simulink subsystem "contact_cana"  (R2024a)
settings: Solver=VariableStepAuto  StartTime=0.0  StopTime=10.0  RelTol=1e-3
libraries: nesl_utility x12, sm_lib x12
settings Model: Creator=Acwa-Remote  LastModifiedBy=VincentPERRET

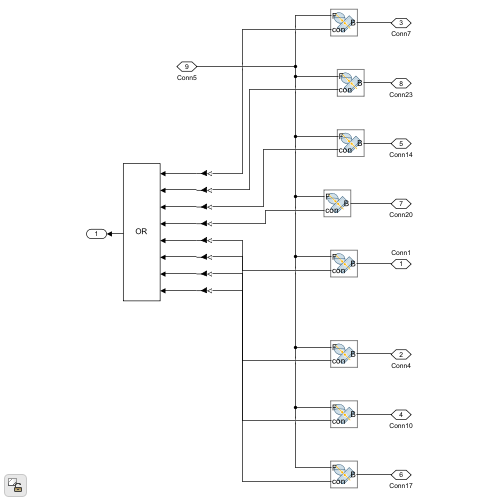
[thumbnail: Simulink's stored preview of the top-level diagram]
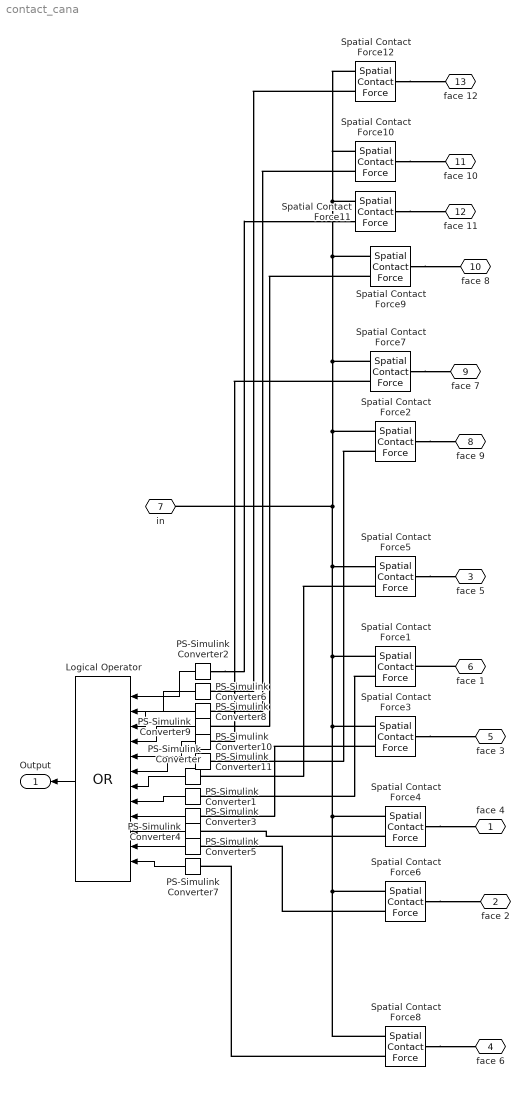
== system contact_cana ==
  Logical Operator : Logic  Operator=OR  Inputs=12  AllPortsSameDT=off  OutDataTypeStr=boolean
  PS-Simulink Converter{,1..11} (12 alike) : nesl_utility/PS-Simulink Converter  PhysicalDomain=network_engine_domain  SubClassName=ps_output  LeftPortType=input  RightPortType=output  PseudoPeriodic=off  Frequencies=[]  VectorFormat=inherit  Unit=inherit  AffineConversion=off
  Spatial Contact Force{1..7,9..12} (11 alike) : sm_lib/Forces and Torques/Spatial Contact Force  NormalForceType=SmoothSpringDamper  NormalStiffness=stiff  NormalStiffnessUnits=N/m  NormalDamping=damp  NormalDampingUnits=N/(m/s)  NormalTransitionRegionWidth=trw  NormalTransitionRegionWidthUnits=mm  FrictionType=SmoothStickSlip  CoefficientOfStaticFriction=cana_fs  CoefficientOfDynamicFriction=cana_fd  FrictionalCriticalVelocity=1e-3  FrictionalCriticalVelocityUnits=m/s  SenseContactSignal=on  SensePenetrationDepth=off  SenseSeparationDistance=off  SenseNormalForceMagnitude=off  SenseFrictionalForceMagnitude=off  SenseNormalVelocity=off  SenseTangentialVelocity=off  SenseContactBaseRotation=off  SenseContactBaseTranslation=off  SenseContactFollowerRotation=off  SenseContactFollowerTranslation=off  ZeroCrossDetectContactStartAndEnd=off
  Spatial Contact Force8 : sm_lib/Forces and Torques/Spatial Contact Force  NormalForceType=SmoothSpringDamper  NormalStiffness=stiff  NormalStiffnessUnits=N/m  NormalDamping=damp  NormalDampingUnits=N/(m/s)  NormalTransitionRegionWidth=trw  NormalTransitionRegionWidthUnits=mm  FrictionType=SmoothStickSlip  CoefficientOfStaticFriction=0.3  CoefficientOfDynamicFriction=0.3  FrictionalCriticalVelocity=1e-3  FrictionalCriticalVelocityUnits=m/s  SenseContactSignal=on  SensePenetrationDepth=off  SenseSeparationDistance=off  SenseNormalForceMagnitude=off  SenseFrictionalForceMagnitude=off  SenseNormalVelocity=off  SenseTangentialVelocity=off  SenseContactBaseRotation=off  SenseContactBaseTranslation=off  SenseContactFollowerRotation=off  SenseContactFollowerTranslation=off  ZeroCrossDetectContactStartAndEnd=off
  face 4 : PMIOPort  Side=Left
  face 2 : PMIOPort  Port=2  Side=Left
  face 5 : PMIOPort  Port=3  Side=Left
  face 6 : PMIOPort  Port=4  Side=Left
  face 3 : PMIOPort  Port=5  Side=Left
  face 1 : PMIOPort  Port=6  Side=Left
  in : PMIOPort  Port=7  Side=Right
  face 9 : PMIOPort  Port=8  Side=Left
  face 7 : PMIOPort  Port=9  Side=Left
  face 8 : PMIOPort  Port=10  Side=Left
  face 10 : PMIOPort  Port=11  Side=Left
  face 11 : PMIOPort  Port=12  Side=Left
  face 12 : PMIOPort  Port=13  Side=Left
  Output : Outport
  wires:
  PS-Simulink Converter/1 -> Logical Operator/7
  PS-Simulink Converter1/1 -> Logical Operator/8
  PS-Simulink Converter3/1 -> Logical Operator/9
  PS-Simulink Converter4/1 -> Logical Operator/10
  PS-Simulink Converter5/1 -> Logical Operator/11
  PS-Simulink Converter7/1 -> Logical Operator/12
  Logical Operator/1 -> Output/1
  PS-Simulink Converter11/1 -> Logical Operator/6
  PS-Simulink Converter10/1 -> Logical Operator/5
  PS-Simulink Converter9/1 -> Logical Operator/4
  PS-Simulink Converter8/1 -> Logical Operator/3
  PS-Simulink Converter6/1 -> Logical Operator/2
  PS-Simulink Converter2/1 -> Logical Operator/1
  connections:
  Spatial Contact Force6/RConn1 -- Spatial Contact Force12/RConn1 -- Spatial Contact Force10/RConn1 -- Spatial Contact Force11/RConn1 -- Spatial Contact Force9/RConn1 -- Spatial Contact Force7/RConn1 -- Spatial Contact Force2/RConn1 -- in/RConn1 -- Spatial Contact Force5/RConn1 -- Spatial Contact Force1/RConn1 -- Spatial Contact Force3/RConn1 -- Spatial Contact Force4/RConn1 -- Spatial Contact Force8/RConn1
  Spatial Contact Force5/RConn2 -- PS-Simulink Converter/LConn1
  face 1/RConn1 -- Spatial Contact Force1/LConn1
  Spatial Contact Force1/RConn2 -- PS-Simulink Converter1/LConn1
  Spatial Contact Force3/RConn2 -- PS-Simulink Converter3/LConn1
  Spatial Contact Force4/RConn2 -- PS-Simulink Converter4/LConn1
  Spatial Contact Force6/RConn2 -- PS-Simulink Converter5/LConn1
  Spatial Contact Force8/RConn2 -- PS-Simulink Converter7/LConn1
  Spatial Contact Force5/LConn1 -- face 5/RConn1
  Spatial Contact Force3/LConn1 -- face 3/RConn1
  Spatial Contact Force4/LConn1 -- face 4/RConn1
  Spatial Contact Force6/LConn1 -- face 2/RConn1
  Spatial Contact Force8/LConn1 -- face 6/RConn1
  Spatial Contact Force2/LConn1 -- face 9/RConn1
  Spatial Contact Force2/RConn2 -- PS-Simulink Converter11/LConn1
  Spatial Contact Force7/LConn1 -- face 7/RConn1
  Spatial Contact Force7/RConn2 -- PS-Simulink Converter10/LConn1
  Spatial Contact Force9/LConn1 -- face 8/RConn1
  Spatial Contact Force9/RConn2 -- PS-Simulink Converter9/LConn1
  Spatial Contact Force10/LConn1 -- face 10/RConn1
  Spatial Contact Force10/RConn2 -- PS-Simulink Converter8/LConn1
  Spatial Contact Force11/LConn1 -- face 11/RConn1
  PS-Simulink Converter2/LConn1 -- Spatial Contact Force11/RConn2
  Spatial Contact Force12/LConn1 -- face 12/RConn1
  Spatial Contact Force12/RConn2 -- PS-Simulink Converter6/LConn1
